simulink model "TSCLAB_ModelPV_21"  (R2020a)
settings: Solver=VariableStepAuto  StartTime=0.0  StopTime=800  RelTol=1e-3
undefined symbols (not defined in the file or in its folder): serial
libraries: instrumentlib x3, simulink x1
settings Model: Creator=vasanza  LastModifiedBy=Familia Zúñiga Vega
settings SolverCC: AlgebraicLoopSolver=LineSearch
settings DebuggingCC: ArithmeticOperatorsInVariantConditions=warning
settings SFSimCC: CustomCodeUndefinedFunction=UseInterfaceOnly

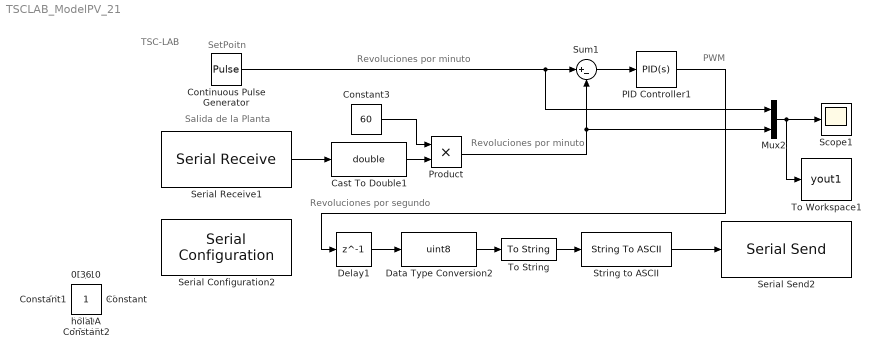
== system TSCLAB_ModelPV_21 ==
  note: PWM
  note: Salida de la Planta
  note: Revoluciones por minuto
  note: Revoluciones por segundo
  note: SetPoitn
  note: TSC-LAB
  note: Revoluciones por minuto
  Cast To Double1 : DataTypeConversion  OutDataTypeStr=double
  Constant3 : Constant  Value=60
  Continuous Pulse Generator : DiscretePulseGenerator  PulseType=Time based  Amplitude=255  Period=26  PulseWidth=50
  Data Type Conversion2 : DataTypeConversion  OutDataTypeStr=uint8
  Delay1 : Delay  DelayLength=1  InitialCondition=0
  Mux2 : Mux  Inputs=2
  PID Controller1 : simulink/Continuous/PID Controller  Controller=PID  Form=Parallel  TimeDomain=Continuous-time  UseExternalTs=off  SampleTime=-1  IntegratorMethod=Forward Euler  FilterMethod=Forward Euler  ControllerParametersSource=internal  P=0.000109  I=0.000416  D=0  UseFilter=on  N=100  TunerSelectOption=Transfer Function Based (PID Tuner App)  InitialConditionSource=internal  InitialConditionForIntegrator=0  InitialConditionForFilter=0  DifferentiatorICPrevScaledInput=0  ExternalReset=none  TrackingMode=off  Kt=1  LimitOutput=on  UpperSaturationLimit=inf  LowerSaturationLimit=0  LinearizeAsGain=on  AntiWindupMode=none  Kb=1  POutMin=[]  POutMax=[]  IOutMin=[]  IOutMax=[]  DOutMin=[]  DOutMax=[]  NOutMin=[]  NOutMax=[]  SumOutMin=[]  SumOutMax=[]  SaturationOutMin=[]  SaturationOutMax=[]  PParamMin=[]  PParamMax=[]  IParamMin=[]  IParamMax=[]  DParamMin=[]  DParamMax=[]  NParamMin=[]  NParamMax=[]  KbParamMin=[]  KbParamMax=[]  KtParamMin=[]  KtParamMax=[]  KbOutMin=[]  KbOutMax=[]  KtOutMin=[]  KtOutMax=[]  IntegratorOutMin=[]  IntegratorOutMax=[]  FilterOutMin=[]  FilterOutMax=[]  SumI1OutMin=[]  SumI1OutMax=[]  SumI2OutMin=[]  SumI2OutMax=[]  SumI3OutMin=[]  SumI3OutMax=[]  SumI4OutMin=[]  SumI4OutMax=[]  SumDOutMin=[]  SumDOutMax=[]  DifferentiatorOutMin=[]  DifferentiatorOutMax=[]  FilterDiffOutCoefMin=[]  FilterDiffOutCoefMax=[]  ReciprocalOutMin=[]  ReciprocalOutMax=[]  SumDenOutMin=[]  SumDenOutMax=[]  SumNumOutMin=[]  SumNumOutMax=[]  DivideOutMin=[]  DivideOutMax=[]  UdiffTsProdOutMin=[]  UdiffTsProdOutMax=[]  NTsProdOutMin=[]  NTsProdOutMax=[]  UintegralTsProdOutMin=[]  UintegralTsProdOutMax=[]  UngainTsProdOutMin=[]  UngainTsProdOutMax=[]  IntegratorContinuousStateAttributes=''  IntegratorStateMustResolveToSignalObject=off  IntegratorRTWStateStorageClass=Auto  FilterContinuousStateAttributes=''  FilterStateMustResolveToSignalObject=off  FilterRTWStateStorageClass=Auto  ParallelPVariant=InternalParameters  IdealPVariant=Disabled  IVariant=InternalParameters  DVariant=InternalParameters  IntegratorVariant=Continuous  SatVariant=Enabled  AWVariant=Passthrough  PCopyVariant=Disabled  TRVariant=Disabled  FdbkBlocksVariant=Forward  IdealPFdbkVariant=Disabled  SatFdbkVariant=Disabled  DerivativeFilterVariant=ContFilter  NVariant=InternalParameters  NCopyVariant=Disabled  FilterICVariant=InternalICsFilter  IntegratorICVariant=InternalICs  ExternalResetVariant=Disabled  TRSumVariant=Passthrough  SumFdbkVariant=Disabled  SumVariant=Sum_PID  TsampFilterVariant=InternalTs  TsampNgainVariant=Passthrough  TsampIntegralVariant=Passthrough
  Product : Product
  Scope1 : Scope
  Serial Configuration2 : instrumentlib/Serial Configuration  Priority=-200000  ComPortMenu=COM30  ComPort=COM30  ObjConstructor=serial('COM30');  BaudRate=115200  DataBits=8  Parity=none  StopBits=1  FlowControl=none  Timeout=200  ByteOrder=LittleEndian
  Serial Receive1 : instrumentlib/Serial Receive  ComPortMenu=COM30  ComPort=COM30  ObjConstructor=serial('COM30');  Terminator=<none>  DataSize=[1 1]  DataType=uint8  EnableBlockingMode=on  ActionDataUnavailable=Output last received value  CustomValue=0  SampleTime=0.999
  Serial Send2 : instrumentlib/Serial Send  ComPortMenu=COM30  ComPort=COM30  ObjConstructor=serial('COM30');  Terminator=<none>  EnableBlockingMode=on
  String to ASCII : StringToASCII
  Sum1 : Sum  Inputs=|+-
  To String : ToString
  To Workspace1 : ToWorkspace  VariableName=yout1  SampleTime=-1
      settings: Save2DSignal=2-D array (concatenate along first dimension)
  $ : Constant  IOType=siggen  Value=36
  , : Constant  IOType=siggen  Value=44
  {0,10,255,311,12345} (5 alike) : Constant  IOType=siggen
  0A : Constant  IOType=siggen  Value=10
  0D : Constant  IOType=siggen  Value=13
  13 : Constant  IOType=siggen  Value=13
  36 : Constant  IOType=siggen  Value=36
  Constant : Constant  IOType=siggen
  Constant1 : Constant  IOType=siggen
  Constant2 : Constant  IOType=siggen
  hola : Constant  IOType=siggen
  wires:
  Cast To Double1/1 -> Product/2
  Product/1 -> Mux2/2, Sum1/2
  Constant3/1 -> Product/1
  Serial Receive1/1 -> Cast To Double1/1
  String to ASCII/1 -> Serial Send2/1
  Continuous Pulse Generator/1 -> Mux2/1, Sum1/1
  Sum1/1 -> PID Controller1/1
  Delay1/1 -> Data Type Conversion2/1
  PID Controller1/1 -> Delay1/1
  Mux2/1 -> To Workspace1/1, Scope1/1
  Data Type Conversion2/1 -> To String/1
  To String/1 -> String to ASCII/1
